simulink model "trial2"  (R2021a)
settings: Solver=VariableStepAuto  StartTime=0.0  StopTime=10.0  RelTol=1e-3
libraries: robotmobilelib x1
settings Model: Creator=templ  LastModifiedBy=templ

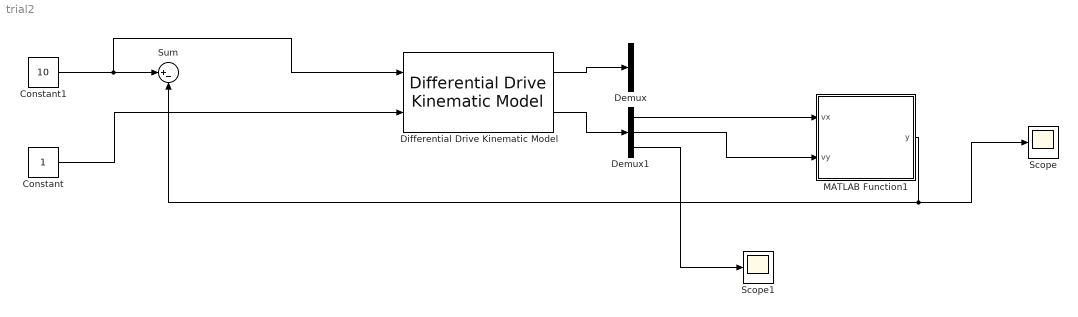
== system trial2 ==
  Constant : Constant
  Constant1 : Constant  Value=10
  Demux : Demux  Outputs=3
  Demux1 : Demux  Outputs=3
  Differential Drive Kinematic Model : robotmobilelib/Differential Drive Kinematic Model  VehicleInputs=Vehicle Speed & Heading Angular Velocity  WheelRadius=0.0105  WheelSpeedRange=[-inf inf]  TrackWidth=0.05  InitialState=[0; 0; 0]  SimulateUsing=Interpreted execution
      settings: SourceProductBaseCode=RO
  MATLAB Function1 : MATLAB Function  TreatAsAtomicUnit=on
  Scope : Scope
  Scope1 : Scope
  Sum : Sum  Inputs=|+-
  wires:
  Differential Drive Kinematic Model/1 -> Demux/1
  Differential Drive Kinematic Model/2 -> Demux1/1
  Demux1/1 -> MATLAB Function1/1(vx)
  Demux1/2 -> MATLAB Function1/2(vy)
  Constant1/1 -> Differential Drive Kinematic Model/1, Sum/1
  MATLAB Function1/1(y) -> Sum/2, Scope/1
  Constant/1 -> Differential Drive Kinematic Model/2
  Demux1/3 -> Scope1/1

== matlab function trial2/MATLAB Function1 ==
  data: vx input; y output; vy input
function y = fcn(vx,vy)
vnet=sqrt((vx^2)+(vy^2));



y = vnet;
